simulink model "pmsm_control_ortega_observer_2010"  (R2021a)
settings: Solver=VariableStepAuto  StartTime=0.0  StopTime=10.0  RelTol=1e-3
libraries: mcbcontrolslib x4, pid_lib x3, simulink x2, eeGeneralControl x1, autolibpmsmexterior x1
settings Model: OrderedModelArguments=off  Creator=Rodrigo  LastModifiedBy=Rodrigo

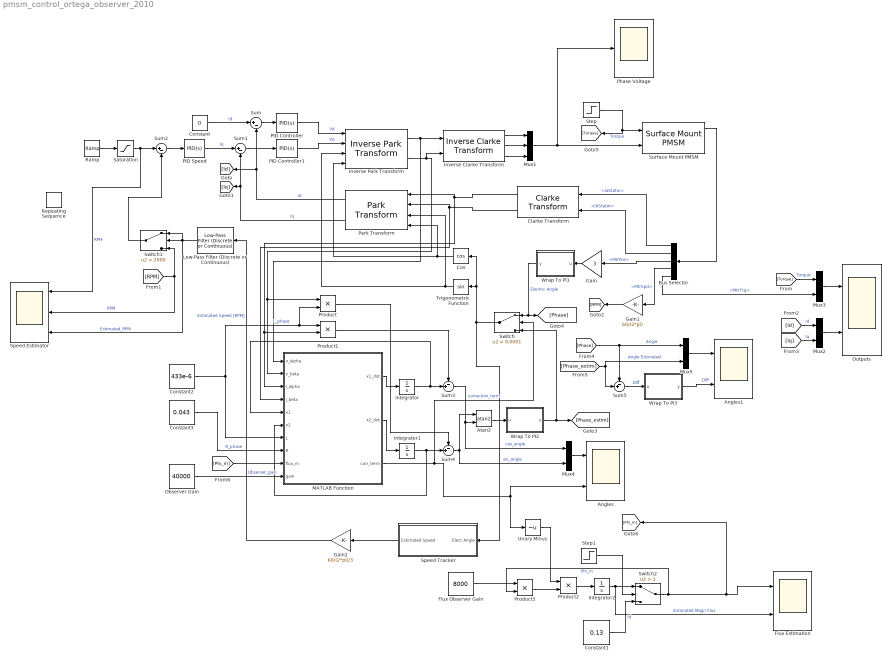
== system pmsm_control_ortega_observer_2010 ==
  Angles : Scope  NumInputPorts=2
  Angles1 : Scope  NumInputPorts=2
  Atan2 : Trigonometry  Operator=atan2
  Bus Selector : BusSelector  OutputSignals=IaStator,IbStator,MtrPos,MtrSpd,MtrTrq
  Clarke Transform : mcbcontrolslib/Clarke Transform  VariantControl=Variant2
  Constant : Constant  Value=0
  Constant1 : Constant  Value=0.13
  Constant2 : Constant  Value=433e-6
  Constant3 : Constant  Value=0.043
  Cos : Trigonometry  Operator=cos
  Flux Estimation : Scope  NumInputPorts=2
  Flux Observer Gain : Constant  Value=8000
  Gain : Gain  Gain=3
  Gain1 : Gain  Gain=60/(2*pi)
  Gain2 : Gain  Gain=60/(2*pi)/3
  Integrator : Integrator
  Integrator1 : Integrator
  Integrator2 : Integrator
  Inverse Clarke Transform : mcbcontrolslib/Inverse Clarke Transform
      settings: SourceProductBaseCode=MT
  Inverse Park Transform : mcbcontrolslib/Inverse Park Transform  AxisAlignment=D-axis
  Low-Pass Filter (Discrete or Continuous) : eeGeneralControl/Low-Pass Filter (Discrete or Continuous)  K=1  T=0.1  B=inf  A=-inf  init_option=Inherited from block input  x0=0  Ts=0
  MATLAB Function : MATLAB Function  TreatAsAtomicUnit=on
  Mux1 : Mux  Inputs=3
  Mux{2..5} (4 alike) : Mux  Inputs=2
  Observer Gain : Constant  Value=40000
  Outputs : Scope  NumInputPorts=2
  PID Controller : pid_lib/PID Controller  Controller=PID  Form=Parallel  TimeDomain=Continuous-time  UseExternalTs=off  SampleTime=-1  IntegratorMethod=Forward Euler  FilterMethod=Forward Euler  ControllerParametersSource=internal  P=0.433  I=43  D=0  UseFilter=on  N=100  TunerSelectOption=Transfer Function Based (PID Tuner App)  InitialConditionSource=internal  InitialConditionForIntegrator=0  InitialConditionForFilter=0  DifferentiatorICPrevScaledInput=0  ExternalReset=none  TrackingMode=off  Kt=1  LimitOutput=off  SatLimitsSource=internal  UpperSaturationLimit=inf  LowerSaturationLimit=-inf  LinearizeAsGain=on  AntiWindupMode=none  Kb=1  POutMin=[]  POutMax=[]  IOutMin=[]  IOutMax=[]  DOutMin=[]  DOutMax=[]  NOutMin=[]  NOutMax=[]  SumOutMin=[]  SumOutMax=[]  SaturationOutMin=[]  SaturationOutMax=[]  PParamMin=[]  PParamMax=[]  IParamMin=[]  IParamMax=[]  DParamMin=[]  DParamMax=[]  NParamMin=[]  NParamMax=[]  KbParamMin=[]  KbParamMax=[]  KtParamMin=[]  KtParamMax=[]  KbOutMin=[]  KbOutMax=[]  KtOutMin=[]  KtOutMax=[]  IntegratorOutMin=[]  IntegratorOutMax=[]  FilterOutMin=[]  FilterOutMax=[]  SumI1OutMin=[]  SumI1OutMax=[]  SumI2OutMin=[]  SumI2OutMax=[]  SumI3OutMin=[]  SumI3OutMax=[]  SumI4OutMin=[]  SumI4OutMax=[]  SumDOutMin=[]  SumDOutMax=[]  DifferentiatorOutMin=[]  DifferentiatorOutMax=[]  FilterDiffOutCoefMin=[]  FilterDiffOutCoefMax=[]  ReciprocalOutMin=[]  ReciprocalOutMax=[]  SumDenOutMin=[]  SumDenOutMax=[]  SumNumOutMin=[]  SumNumOutMax=[]  DivideOutMin=[]  DivideOutMax=[]  UdiffTsProdOutMin=[]  UdiffTsProdOutMax=[]  NTsProdOutMin=[]  NTsProdOutMax=[]  UintegralTsProdOutMin=[]  UintegralTsProdOutMax=[]  UngainTsProdOutMin=[]  UngainTsProdOutMax=[]  IntegratorContinuousStateAttributes=''  IntegratorStateMustResolveToSignalObject=off  IntegratorRTWStateStorageClass=Auto  FilterContinuousStateAttributes=''  FilterStateMustResolveToSignalObject=off  FilterRTWStateStorageClass=Auto  ParallelPVariant=InternalParameters  IdealPVariant=Disabled  IVariant=InternalParameters  DVariant=InternalParameters  IntegratorVariant=Continuous  SatVariant=Disabled  AWVariant=Passthrough  PCopyVariant=Disabled  TRVariant=Disabled  FdbkBlocksVariant=Forward  IdealPFdbkVariant=Disabled  SatFdbkVariant=Disabled  DerivativeFilterVariant=ContFilter  NVariant=InternalParameters  NCopyVariant=Disabled  FilterICVariant=InternalICsFilter  IntegratorICVariant=InternalICs  ExternalResetVariant=Disabled  TRSumVariant=Passthrough  SumFdbkVariant=Disabled  SumVariant=Sum_PID  TsampFilterVariant=InternalTs  TsampNgainVariant=Passthrough  TsampIntegralVariant=Passthrough  ExternalSaturationOutDataTypeStr=Inherit: Same as second input
  PID Controller1 : pid_lib/PID Controller  Controller=PID  Form=Parallel  TimeDomain=Continuous-time  UseExternalTs=off  SampleTime=-1  IntegratorMethod=Forward Euler  FilterMethod=Forward Euler  ControllerParametersSource=internal  P=0.433  I=43  D=0  UseFilter=on  N=100  TunerSelectOption=Transfer Function Based (PID Tuner App)  InitialConditionSource=internal  InitialConditionForIntegrator=0  InitialConditionForFilter=0  DifferentiatorICPrevScaledInput=0  ExternalReset=none  TrackingMode=off  Kt=1  LimitOutput=off  SatLimitsSource=internal  UpperSaturationLimit=inf  LowerSaturationLimit=-inf  LinearizeAsGain=on  AntiWindupMode=none  Kb=1  POutMin=[]  POutMax=[]  IOutMin=[]  IOutMax=[]  DOutMin=[]  DOutMax=[]  NOutMin=[]  NOutMax=[]  SumOutMin=[]  SumOutMax=[]  SaturationOutMin=[]  SaturationOutMax=[]  PParamMin=[]  PParamMax=[]  IParamMin=[]  IParamMax=[]  DParamMin=[]  DParamMax=[]  NParamMin=[]  NParamMax=[]  KbParamMin=[]  KbParamMax=[]  KtParamMin=[]  KtParamMax=[]  KbOutMin=[]  KbOutMax=[]  KtOutMin=[]  KtOutMax=[]  IntegratorOutMin=[]  IntegratorOutMax=[]  FilterOutMin=[]  FilterOutMax=[]  SumI1OutMin=[]  SumI1OutMax=[]  SumI2OutMin=[]  SumI2OutMax=[]  SumI3OutMin=[]  SumI3OutMax=[]  SumI4OutMin=[]  SumI4OutMax=[]  SumDOutMin=[]  SumDOutMax=[]  DifferentiatorOutMin=[]  DifferentiatorOutMax=[]  FilterDiffOutCoefMin=[]  FilterDiffOutCoefMax=[]  ReciprocalOutMin=[]  ReciprocalOutMax=[]  SumDenOutMin=[]  SumDenOutMax=[]  SumNumOutMin=[]  SumNumOutMax=[]  DivideOutMin=[]  DivideOutMax=[]  UdiffTsProdOutMin=[]  UdiffTsProdOutMax=[]  NTsProdOutMin=[]  NTsProdOutMax=[]  UintegralTsProdOutMin=[]  UintegralTsProdOutMax=[]  UngainTsProdOutMin=[]  UngainTsProdOutMax=[]  IntegratorContinuousStateAttributes=''  IntegratorStateMustResolveToSignalObject=off  IntegratorRTWStateStorageClass=Auto  FilterContinuousStateAttributes=''  FilterStateMustResolveToSignalObject=off  FilterRTWStateStorageClass=Auto  ParallelPVariant=InternalParameters  IdealPVariant=Disabled  IVariant=InternalParameters  DVariant=InternalParameters  IntegratorVariant=Continuous  SatVariant=Disabled  AWVariant=Passthrough  PCopyVariant=Disabled  TRVariant=Disabled  FdbkBlocksVariant=Forward  IdealPFdbkVariant=Disabled  SatFdbkVariant=Disabled  DerivativeFilterVariant=ContFilter  NVariant=InternalParameters  NCopyVariant=Disabled  FilterICVariant=InternalICsFilter  IntegratorICVariant=InternalICs  ExternalResetVariant=Disabled  TRSumVariant=Passthrough  SumFdbkVariant=Disabled  SumVariant=Sum_PID  TsampFilterVariant=InternalTs  TsampNgainVariant=Passthrough  TsampIntegralVariant=Passthrough  ExternalSaturationOutDataTypeStr=Inherit: Same as second input
  PID Speed : pid_lib/PID Controller  Controller=PID  Form=Parallel  TimeDomain=Continuous-time  UseExternalTs=off  SampleTime=-1  IntegratorMethod=Forward Euler  FilterMethod=Forward Euler  ControllerParametersSource=internal  P=0.07  I=0.04  D=0.02  UseFilter=on  N=50  TunerSelectOption=Transfer Function Based (PID Tuner App)  InitialConditionSource=internal  InitialConditionForIntegrator=0  InitialConditionForFilter=0  DifferentiatorICPrevScaledInput=0  ExternalReset=none  TrackingMode=off  Kt=1  LimitOutput=off  SatLimitsSource=internal  UpperSaturationLimit=inf  LowerSaturationLimit=-inf  LinearizeAsGain=on  AntiWindupMode=none  Kb=1  POutMin=[]  POutMax=[]  IOutMin=[]  IOutMax=[]  DOutMin=[]  DOutMax=[]  NOutMin=[]  NOutMax=[]  SumOutMin=[]  SumOutMax=[]  SaturationOutMin=[]  SaturationOutMax=[]  PParamMin=[]  PParamMax=[]  IParamMin=[]  IParamMax=[]  DParamMin=[]  DParamMax=[]  NParamMin=[]  NParamMax=[]  KbParamMin=[]  KbParamMax=[]  KtParamMin=[]  KtParamMax=[]  KbOutMin=[]  KbOutMax=[]  KtOutMin=[]  KtOutMax=[]  IntegratorOutMin=[]  IntegratorOutMax=[]  FilterOutMin=[]  FilterOutMax=[]  SumI1OutMin=[]  SumI1OutMax=[]  SumI2OutMin=[]  SumI2OutMax=[]  SumI3OutMin=[]  SumI3OutMax=[]  SumI4OutMin=[]  SumI4OutMax=[]  SumDOutMin=[]  SumDOutMax=[]  DifferentiatorOutMin=[]  DifferentiatorOutMax=[]  FilterDiffOutCoefMin=[]  FilterDiffOutCoefMax=[]  ReciprocalOutMin=[]  ReciprocalOutMax=[]  SumDenOutMin=[]  SumDenOutMax=[]  SumNumOutMin=[]  SumNumOutMax=[]  DivideOutMin=[]  DivideOutMax=[]  UdiffTsProdOutMin=[]  UdiffTsProdOutMax=[]  NTsProdOutMin=[]  NTsProdOutMax=[]  UintegralTsProdOutMin=[]  UintegralTsProdOutMax=[]  UngainTsProdOutMin=[]  UngainTsProdOutMax=[]  IntegratorContinuousStateAttributes=''  IntegratorStateMustResolveToSignalObject=off  IntegratorRTWStateStorageClass=Auto  FilterContinuousStateAttributes=''  FilterStateMustResolveToSignalObject=off  FilterRTWStateStorageClass=Auto  ParallelPVariant=InternalParameters  IdealPVariant=Disabled  IVariant=InternalParameters  DVariant=InternalParameters  IntegratorVariant=Continuous  SatVariant=Disabled  AWVariant=Passthrough  PCopyVariant=Disabled  TRVariant=Disabled  FdbkBlocksVariant=Forward  IdealPFdbkVariant=Disabled  SatFdbkVariant=Disabled  DerivativeFilterVariant=ContFilter  NVariant=InternalParameters  NCopyVariant=Disabled  FilterICVariant=InternalICsFilter  IntegratorICVariant=InternalICs  ExternalResetVariant=Disabled  TRSumVariant=Passthrough  SumFdbkVariant=Disabled  SumVariant=Sum_PID  TsampFilterVariant=InternalTs  TsampNgainVariant=Passthrough  TsampIntegralVariant=Passthrough  ExternalSaturationOutDataTypeStr=Inherit: Same as second input
  Park Transform : mcbcontrolslib/Park Transform  AxisAlignment=D-axis
      settings: SourceProductBaseCode=MT
  Phase Voltage : Scope
  Product{,1..3} (4 alike) : Product
  Ramp : simulink/Sources/Ramp  slope=200  start=0  InitialOutput=0
  Repeating Sequence : simulink/Sources/Repeating Sequence  rep_seq_t=[0 1 3 4 6 7]  rep_seq_y=[0 600 600 -600 -600 600]
  Saturation : Saturate  UpperLimit=500  LowerLimit=-500
  Speed Estimator : Scope  NumInputPorts=3
  Speed Tracker : Subsystem
  Step : Step  Time=5  After=10  SampleTime=0
  Step1 : Step  After=2  SampleTime=0
  Sum : Sum  Inputs=|+-
  Sum1 : Sum  Inputs=|+-
  Sum2 : Sum  Inputs=|+-
  Sum3 : Sum  Inputs=-+|
  Sum4 : Sum  Inputs=-+|
  Sum5 : Sum  Inputs=-+|
  Surface Mount PMSM : autolibpmsmexterior/Surface Mount PMSM  port_config=Torque  sim_type=Continuous  Ts=0.001  P=3  Rs=0.0433  Ldq_=436e-6  KConstText=Permanent flux linkage constant (lambda_pm):  lambda_pm=0.146  Ke=159.9771  Kt=1.323  mechanical=[0.20, 4.924e-4, 0]  idq0=[0 0]  theta_init=0  omega_init=0  KConst=0.146  lambda_pm_calc=0.146  RefBlkName='autolibpmsmexterior/Surface Mount PMSM'  aMode=5  Ldq="[0.0017      0.0017]"
      settings: SourceProductBaseCode=PW,DR,MT,UV,VE
  Switch : Switch  Criteria=u2 > Threshold  Threshold=0.0001
  Switch1 : Switch  Criteria=u2 > Threshold  Threshold=2000
  Switch2 : Switch  Criteria=u2 > Threshold  Threshold=1
  Trigonometric Function : Trigonometry
  Unary Minus : UnaryMinus
  Wrap To PI1 : MATLAB Function  TreatAsAtomicUnit=on
  Wrap To PI2 : MATLAB Function  TreatAsAtomicUnit=on
  Wrap To PI3 : MATLAB Function  TreatAsAtomicUnit=on
  wires:
  Inverse Clarke Transform/1 -> Mux1/1
  Inverse Clarke Transform/2 -> Mux1/2
  Inverse Clarke Transform/3 -> Mux1/3
  Mux1/1 -> Surface Mount PMSM/2, Phase Voltage/1
  Inverse Park Transform/1 -> Inverse Clarke Transform/1, MATLAB Function/1(v_alpha)
  Inverse Park Transform/2 -> Inverse Clarke Transform/2, MATLAB Function/2(v_beta), Product/1
  Clarke Transform/1 -> Product1/2, MATLAB Function/3(i_alpha), Park Transform/1
  Clarke Transform/2 -> MATLAB Function/4(i_beta), Park Transform/2
  PID Controller/1 -> Inverse Park Transform/1  "Vd"
  PID Controller1/1 -> Inverse Park Transform/2  "Vq"
  Sum/1 -> PID Controller/1
  Sum1/1 -> PID Controller1/1
  Park Transform/1 -> [Id], Sum/2  "Id"
  Park Transform/2 -> [Iq], Sum1/2  "Iq"
  Step/1 -> [Torque], Surface Mount PMSM/1  "Torque"
  PID Speed/1 -> Sum1/1  "Iq"
  Constant/1 -> Sum/1  "Id"
  Cos/1 -> Park Transform/4, Inverse Park Transform/4
  Trigonometric Function/1 -> Park Transform/3, Inverse Park Transform/3
  Surface Mount PMSM/1 -> Bus Selector/1
  Bus Selector/3 -> Gain/1  "<MtrPos>"
  Bus Selector/1 -> Clarke Transform/1  "<IaStator>"
  Bus Selector/2 -> Clarke Transform/2  "<IbStator>"
  Bus Selector/4 -> Gain1/1  "<MtrSpd>"
  Sum2/1 -> PID Speed/1
  Saturation/1 -> Sum2/1, Speed Estimator/1  "RPM"
  Gain2/1 -> Low-Pass Filter (Discrete or Continuous)/1  "Estimated Speed [RPM]"
  Speed Tracker/1(Estimated Speed) -> Gain2/1
  Observer Gain/1 -> MATLAB Function/10(gain)  "Observer_gain"
  Constant3/1 -> MATLAB Function/8(R)  "R_phase"
  Constant2/1 -> MATLAB Function/7(L), Product/2, Product1/1  "L_phase"
  MATLAB Function/2(x2_dot) -> Integrator1/1
  MATLAB Function/1(x1_dot) -> Integrator/1
  Integrator/1 -> Sum3/2, MATLAB Function/5(x1)
  Integrator1/1 -> Sum4/2, MATLAB Function/6(x2)
  Product1/1 -> Sum3/1
  Sum3/1 -> Mux4/1, Atan2/2  "cos_angle"
  Product/1 -> Sum4/1
  Sum4/1 -> Mux4/2, Atan2/1  "sin_angle"
  Gain/1 -> Wrap To PI1/1(u)
  Wrap To PI1/1(y) -> [Phase], Switch/1  "Electric Angle"
  Switch/1 -> Trigonometric Function/1, Cos/1, Speed Tracker/1(Elect Angle)
  Atan2/1 -> Wrap To PI2/1(u)
  Wrap To PI2/1(y) -> [Phase_estim], Switch/3
  MATLAB Function/3(corr_term) -> Switch/2, Angles/2, Unary Minus/1  "correction_term"
  Low-Pass Filter (Discrete or Continuous)/1 -> Speed Estimator/3, Switch1/1, Switch1/2  "Estimated_RPM"
  Switch1/1 -> Sum2/2
  Gain1/1 -> [RPM]
  [RPM] -> Speed Estimator/2, Switch1/3  "RPM"
  [Torque] -> Mux3/1  "Torque"
  [Iq] -> Mux2/2  "Iq"
  [Id] -> Mux2/1  "Id"
  Product2/1 -> Integrator2/1
  Product3/1 -> Product2/2
  Flux Observer Gain/1 -> Product3/1
  [Phi_m] -> MATLAB Function/9(flux_m)
  Switch2/1 -> [Phi_m], Flux Estimation/1, Product3/2  "Phi_m"
  Step1/1 -> Switch2/2
  Constant1/1 -> Switch2/3  "Id"
  Integrator2/1 -> Flux Estimation/2, Switch2/1  "Estimated Magn Flux"
  Unary Minus/1 -> Product2/1
  [Phase_estim] -> Sum5/2, Mux5/2  "Angle Estimated"
  [Phase] -> Mux5/1, Sum5/1  "Angle"
  Sum5/1 -> Wrap To PI3/1(u)  "Diff"
  Wrap To PI3/1(y) -> Angles1/2  "Diff"
  Bus Selector/5 -> Mux3/2  "<MtrTrq>"
  Mux3/1 -> Outputs/1
  Mux2/1 -> Outputs/2
  Ramp/1 -> Saturation/1
  Mux4/1 -> Angles/1
  Mux5/1 -> Angles1/1

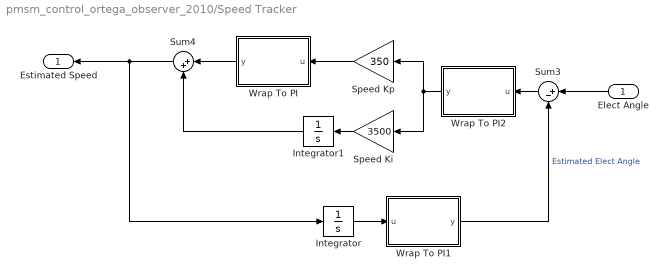
== system pmsm_control_ortega_observer_2010/Speed Tracker ==
  Elect Angle : Inport
  Integrator : Integrator
  Integrator1 : Integrator
  Speed Ki : Gain  Gain=3500
  Speed Kp : Gain  Gain=350
  Sum3 : Sum  Inputs=|+-
  Sum4 : Sum  Inputs=|++
  Wrap To PI : MATLAB Function  TreatAsAtomicUnit=on
  Wrap To PI1 : MATLAB Function  TreatAsAtomicUnit=on
  Wrap To PI2 : MATLAB Function  TreatAsAtomicUnit=on
  Estimated Speed : Outport
  wires:
  Speed Ki/1 -> Integrator1/1
  Integrator1/1 -> Sum4/2
  Sum4/1 -> Estimated Speed/1, Integrator/1
  Integrator/1 -> Wrap To PI1/1(u)
  Wrap To PI/1(y) -> Sum4/1
  Speed Kp/1 -> Wrap To PI/1(u)
  Wrap To PI1/1(y) -> Sum3/2  "Estimated Elect Angle"
  Elect Angle/1 -> Sum3/1
  Sum3/1 -> Wrap To PI2/1(u)
  Wrap To PI2/1(y) -> Speed Kp/1, Speed Ki/1

== matlab function pmsm_control_ortega_observer_2010/Speed Tracker/Wrap To PI1 ==
  data: u input; y output
function y = fcn(u)

y = wrapToPi(u);

== matlab function pmsm_control_ortega_observer_2010/Speed Tracker/Wrap To PI ==
  data: u input; y output
function y = fcn(u)

y = wrapToPi(u);

== matlab function pmsm_control_ortega_observer_2010/MATLAB Function ==
  data: v_alpha input; x1_dot output; v_beta input; i_alpha input; i_beta input; x2_dot output; x1 input; x2 input; L input; R input; flux_m input; gain input; corr_term output
function [x1_dot,x2_dot,corr_term] = ortega_obs(v_alpha, v_beta, i_alpha, i_beta, x1, x2, L, R, flux_m, gain)

corr_term = flux_m^2 - ((x1 - L*i_alpha)^2 + (x2 - L*i_beta)^2);

% if(corr_term < 0)
%      corr_term = 0;
% end

%L = 3/2 * L;
%R = 3/2 * R;
x1_dot = v_alpha - R*i_alpha + gain/2 * (x1 - L*i_alpha) * corr_term;
x2_dot = v_beta - R*i_beta + gain/2 * (x2 - L*i_beta) * corr_term;

%x1 = x1_dot * dt;
%x2 = x2_dot * dt;

%phase = atan2(x2-L*i_beta,x1-L*i_alpha);

== matlab function pmsm_control_ortega_observer_2010/Wrap To PI1 ==
  data: u input; y output
function y = fcn(u)

y = wrapToPi(u);

== matlab function pmsm_control_ortega_observer_2010/Wrap To PI2 ==
  data: u input; y output
function y = fcn(u)

y = wrapToPi(u);

== matlab function pmsm_control_ortega_observer_2010/Speed Tracker/Wrap To PI2 ==
  data: u input; y output
function y = fcn(u)

y = wrapToPi(u);

== matlab function pmsm_control_ortega_observer_2010/Wrap To PI3 ==
  data: u input; y output
function y = fcn(u)

y = wrapToPi(u);
